simulink model "swing_up_test"  (R2020b)
settings: Solver=FixedStepDiscrete  StartTime=0.0  StopTime=Inf  FixedStep=0.001  MaxStep=0.001  RelTol=1e-3  EnableMultiTasking=on
values from neighbouring files (symbols this model uses):
  alfaBest = sin(2*pi*tacc/Tperiod)    [demo.m]    (also in pendulo_modelo.m)
  Xmax = 0.02    [demo.m]    (also in pendulo_modelo.m = 0.045)
  Xmin = -0.02    [demo.m]    (also in pendulo_modelo.m = -0.045)
libraries: simulink x3, arduinolib x2
settings Model: SILPILModeSetting=veronly  ExtModeTrigDuration=2  Creator=aleca  LastModifiedBy=aleca
settings OptimizationCC: EnhancedBackFolding=on  PassReuseOutputArgsAs=Individual arguments  ZeroExternalMemoryAtStartup=off  ZeroInternalMemoryAtStartup=off  MaxStackSize=64  OptimizeBlockOrder=speed  DifferentSizesBufferReuse=on  OptimizationCustomize=off  EfficientTunableParamExpr=on
settings DebuggingCC: ParameterTunabilityLossMsg=error
settings HardwareCC: ProdBitPerInt=16  ProdBitPerPointer=16  ProdBitPerSizeT=16  ProdBitPerPtrDiffT=16  ProdLargestAtomicFloat=None  ProdWordSize=8  ProdHWDeviceType=Atmel->AVR  UseEmbeddedCoderFeatures=off  UseSimulinkCoderFeatures=off
settings SFSimCC: MATLABDynamicMemAlloc=off
settings RTWCC: Description=Embedded Coder  SystemTargetFile=ert.tlc  HardwareBoard=Arduino Mega 2560  TemplateMakefile=ert_default_tmf  Toolchain=Arduino AVR  BuildConfiguration=Faster Runs
settings CodeAppCC: ForceParamTrailComments=on  IgnoreCustomStorageClasses=off  OperatorAnnotations=on  SimulinkDataObjDesc=on  SFDataObjDesc=on  InsertBlockDesc=on
settings ERTTargetCC: SupportContinuousTime=on  SupportNonInlinedSFcns=on  SupportVariableSizeSignals=on  ExtModeStaticAllocSize=2048

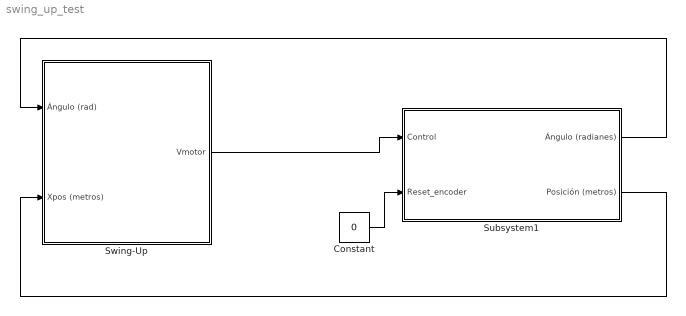
== system swing_up_test ==
  Constant : Constant  Value=0  OutDataTypeStr=boolean  SampleTime=-1
  Subsystem1 : Subsystem
  Swing-Up : Subsystem
  wires:
  Subsystem1/1(Ángulo (radianes)) -> Swing-Up/1(Ángulo (rad))
  Subsystem1/2(Posición (metros)) -> Swing-Up/2(Xpos (metros))
  Swing-Up/1(Vmotor) -> Subsystem1/1(Control)
  Constant/1 -> Subsystem1/2(Reset_encoder)

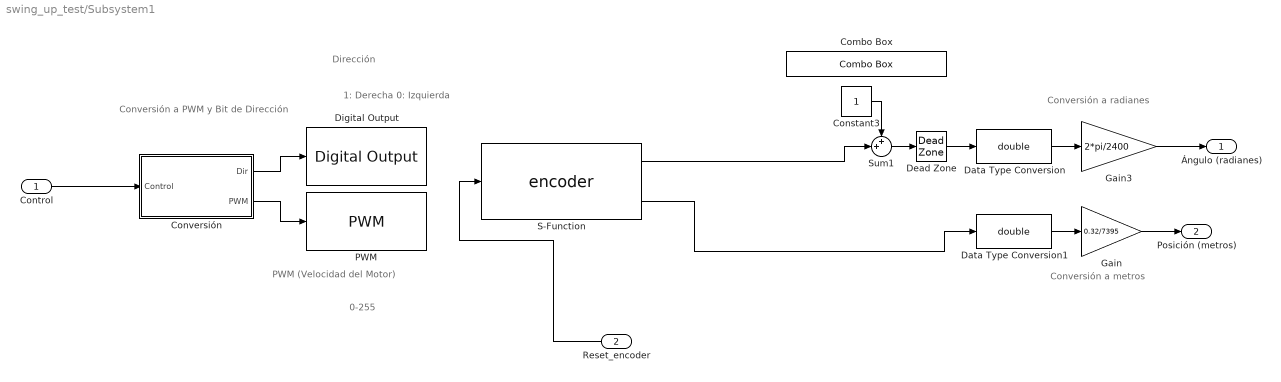
== system swing_up_test/Subsystem1 ==
  note: Conversión a metros
  note: Dirección
  note: PWM (Velocidad del Motor)
  note: 1: Derecha
      | 0: Izquierda
  note: Conversión a radianes
  note: 0-255
  note: Conversión a PWM y
      | Bit de Dirección
  Control : Inport
  Reset_encoder : Inport  Port=2
  Combo Box : ComboBox  LabelPosition=Hide  SelectedLabel=1
      settings: Values={{'0', '1', '2', '-2', '-1'}, [0 1 2 -2 -1]}
  Constant3 : Constant  SampleTime=-1
  Conversión : Subsystem
  Data Type Conversion : DataTypeConversion  OutDataTypeStr=double
  Data Type Conversion1 : DataTypeConversion  OutDataTypeStr=double
  Dead Zone : DeadZone  LowerValue=0  UpperValue=0  SaturateOnIntegerOverflow=on
  Digital Output : arduinolib/Digital Output  pinNumber=10  Direction=output  blockPlatform=arduino
  Gain : Gain  Gain=0.32/7395
  Gain3 : Gain  Gain=2*pi/2400
  PWM : arduinolib/PWM  pinNumber=9  frequencyType=Default  desiredFrequency=490.2  achievableFrequency=490.2
  S-Function : S-Function  FunctionName=encoder  SFunctionModules='encoder_wrapper'  SFunctionDeploymentMode=off  EnableBusSupport=off
  Sum1 : Sum  Inputs=++|
  Ángulo (radianes) : Outport
  Posición (metros) : Outport  Port=2
  wires:
  Gain/1 -> Posición (metros)/1
  Sum1/1 -> Dead Zone/1
  Conversión/1(Dir) -> Digital Output/1
  Conversión/2(PWM) -> PWM/1
  Dead Zone/1 -> Data Type Conversion/1
  Data Type Conversion/1 -> Gain3/1
  Constant3/1 -> Sum1/1
  S-Function/2 -> Data Type Conversion1/1
  Data Type Conversion1/1 -> Gain/1
  Reset_encoder/1 -> S-Function/1
  Control/1 -> Conversión/1(Control)
  Gain3/1 -> Ángulo (radianes)/1
  S-Function/1 -> Sum1/2

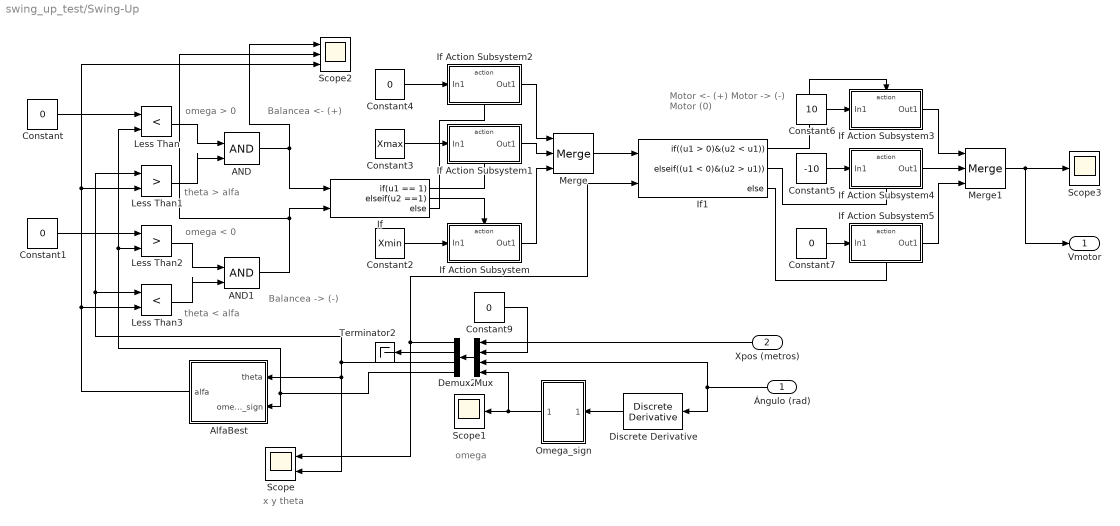
== system swing_up_test/Swing-Up ==
  note: x y theta
  note: omega
  note: Motor <- (+)
      | Motor -> (-)
      | Motor (0)
  note: Balancea -> (-)
  note: theta > alfa
  note: omega > 0
  note: omega < 0
  note: theta < alfa
  note: Balancea <- (+)
  Ángulo (rad) : Inport
  Xpos (metros) : Inport  Port=2
  AND : Logic  IconShape=distinctive  AllPortsSameDT=off  OutDataTypeStr=boolean
  AND1 : Logic  IconShape=distinctive  AllPortsSameDT=off  OutDataTypeStr=boolean
  AlfaBest : Subsystem
      settings: PortSchema="{\"entries\":[{\"content\":{\"sides\":[{\"content\":{\"connectorIds\":[\"Out1\"]},\"type\":\"ConnectorPlacement.EquallySpacedRectSide\",\"uuid\":\"f269d330-2dbf-4a03-aae2-9d91e46d5f46\"},{\"content\":{\"connectorIds\":[\"In1\",\"In2\"],\"side\":\"RIGHT\"},\"type\":\"ConnectorPlacement.EquallySpacedRectSide\",\"uuid\":\"83605d16-f426-4f00-b326-dfdad5d6c839\"},{\"content\":{\"connectorIds\":[],\"side\":\"TOP\"},\"type\":\"ConnectorPlacement.EquallySpacedRectSide\",\"uuid\":\"8003ed59-a4ef-474d-85bb-f26d1ffabd7e\"},{\"content\":{\"connectorIds\":[],\"side\":\"HIDDEN\"},\"type\":\"ConnectorPlacement.EquallySpacedRectSide\",\"uuid\":\"ae6ea9e2-c2fb-4e9e-9ec9-1e561a8d4724\"}]},\"type\":\"ConnectorPlacement.EquallySpacedConnector\",\"uuid\":\"f5174008-485c-4d77-9a7a-ef1ea74262ea\"}],\"packageUris\":[\"http://schema.mathworks.com/mf0/Connector/R2020b\"],\"version\":\"1.0\"}"
  Constant{,1,4,7} (4 alike) : Constant  Value=0  SampleTime=-1
  Constant2 : Constant  Value=Xmin  SampleTime=-1
  Constant3 : Constant  Value=Xmax  SampleTime=-1
  Constant5 : Constant  Value=-10  SampleTime=-1
  Constant6 : Constant  Value=10  SampleTime=-1
  Constant9 : Constant  Value=0
  Demux2 : Demux
  Discrete Derivative : simulink/Discrete/Discrete Derivative  gainval=1.0  ICPrevScaledInput=0.0  OutMin=[]  OutMax=[]  OutDataType=fixdt(1, 16)  OutScaling=2^-10  DoSatur=off
  If : If  NumInputs=2  IfExpression=u1 == 1  ElseIfExpressions=u2 ==1
  If Action Subsystem : Subsystem  TreatAsAtomicUnit=on
  If Action Subsystem1 : Subsystem  TreatAsAtomicUnit=on
  If Action Subsystem2 : Subsystem  TreatAsAtomicUnit=on
  If Action Subsystem3 : Subsystem  TreatAsAtomicUnit=on
  If Action Subsystem4 : Subsystem  TreatAsAtomicUnit=on
  If Action Subsystem5 : Subsystem  TreatAsAtomicUnit=on
  If1 : If  NumInputs=2  IfExpression=(u1 > 0)&(u2 < u1)  ElseIfExpressions=(u1 < 0)&(u2 > u1)
  Less Than : RelationalOperator  Operator=<  OutDataTypeStr=boolean  RndMeth=Simplest
  Less Than1 : RelationalOperator  Operator=>  OutDataTypeStr=boolean  RndMeth=Simplest
  Less Than2 : RelationalOperator  Operator=>  OutDataTypeStr=boolean  RndMeth=Simplest
  Less Than3 : RelationalOperator  Operator=<  OutDataTypeStr=boolean  RndMeth=Simplest
  Merge : Merge  Inputs=3
  Merge1 : Merge  Inputs=3
  Mux : Mux
  Omega_sign : Subsystem
  Scope : Scope  NumInputPorts=2
  Scope1 : Scope
  Scope2 : Scope  NumInputPorts=3
  Scope3 : Scope
  Terminator2 : Terminator
  Vmotor : Outport
  wires:
  Constant3/1 -> If Action Subsystem1/1(In1)
  Less Than1/1 -> AND/2
  AND1/1 -> If/2, Scope2/2
  Omega_sign/1(Out1) -> Scope1/1, Mux/4
  Less Than/1 -> AND/1
  If Action Subsystem5/1(Out1) -> Merge1/3
  Constant1/1 -> Less Than2/1
  Less Than2/1 -> AND1/1
  Constant/1 -> Less Than/1
  If Action Subsystem3/1(Out1) -> Merge1/1
  AND/1 -> Scope2/1, If/1
  Demux2/3 -> AlfaBest/1(theta), Scope/2, Less Than3/1, Less Than1/1
  Mux/1 -> Demux2/1
  If1/1 -> If Action Subsystem3/Action
  If Action Subsystem2/1(Out1) -> Merge/1
  Constant4/1 -> If Action Subsystem2/1(In1)
  Less Than3/1 -> AND1/2
  AlfaBest/1(alfa) -> Scope2/3, Less Than1/2, Less Than3/2
  Constant5/1 -> If Action Subsystem4/1(In1)
  Constant9/1 -> Mux/2
  Demux2/2 -> Terminator2/1
  Ángulo (rad)/1 -> Mux/3, Discrete Derivative/1
  Demux2/4 -> Less Than/2, Less Than2/2, AlfaBest/2(omega_sign)
  Demux2/1 -> Scope/1, If1/2
  Constant7/1 -> If Action Subsystem5/1(In1)
  If/2 -> If Action Subsystem/Action
  Constant2/1 -> If Action Subsystem/1(In1)
  Merge1/1 -> Vmotor/1, Scope3/1
  Constant6/1 -> If Action Subsystem3/1(In1)
  If1/3 -> If Action Subsystem5/Action
  If Action Subsystem/1(Out1) -> Merge/3
  If Action Subsystem4/1(Out1) -> Merge1/2
  Merge/1 -> If1/1
  Discrete Derivative/1 -> Omega_sign/1(In1)
  If/1 -> If Action Subsystem1/Action
  If/3 -> If Action Subsystem2/Action
  If Action Subsystem1/1(Out1) -> Merge/2
  If1/2 -> If Action Subsystem4/Action
  Xpos (metros)/1 -> Mux/1

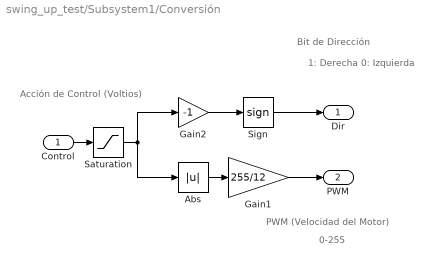
== system swing_up_test/Subsystem1/Conversión ==
  note: Acción de Control
      | (Voltios)
  note: Bit de Dirección
  note: 1: Derecha
      | 0: Izquierda
  note: 0-255
  note: PWM (Velocidad del Motor)
  Control : Inport
  Abs : Abs
  Gain1 : Gain  Gain=255/12
  Gain2 : Gain  Gain=-1
  Saturation : Saturate  UpperLimit=12  LowerLimit=-12
  Sign : Signum
  Dir : Outport
  PWM : Outport  Port=2
  wires:
  Abs/1 -> Gain1/1
  Gain1/1 -> PWM/1
  Control/1 -> Saturation/1
  Saturation/1 -> Gain2/1, Abs/1
  Sign/1 -> Dir/1
  Gain2/1 -> Sign/1

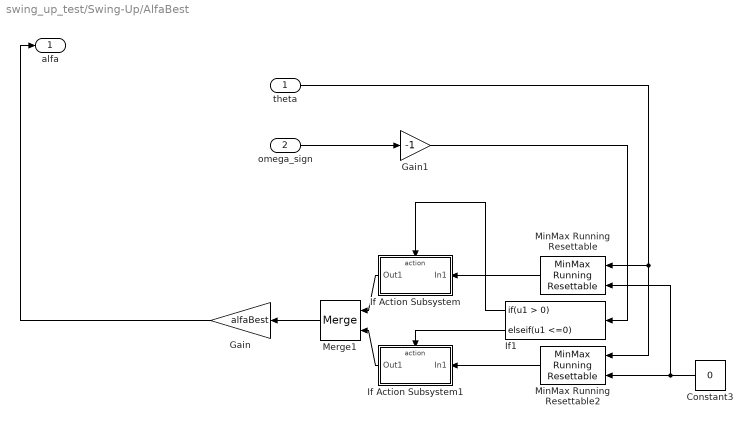
== system swing_up_test/Swing-Up/AlfaBest ==
  theta : Inport
  omega_sign : Inport  Port=2
  Constant3 : Constant  Value=0
  Gain : Gain  Gain=alfaBest
  Gain1 : Gain  Gain=-1
  If Action Subsystem : Subsystem  TreatAsAtomicUnit=on
  If Action Subsystem1 : Subsystem  TreatAsAtomicUnit=on
  If1 : If  ElseIfExpressions=u1 <=0  ShowElse=off
  Merge1 : Merge
  MinMax Running Resettable : simulink/Math Operations/MinMax Running Resettable  Function=max  vinit=0.0
  MinMax Running Resettable2 : simulink/Math Operations/MinMax Running Resettable  Function=min  vinit=0.0
  alfa : Outport
  wires:
  Constant3/1 -> MinMax Running Resettable/2, MinMax Running Resettable2/2
  If Action Subsystem1/1(Out1) -> Merge1/2
  theta/1 -> MinMax Running Resettable2/1, MinMax Running Resettable/1
  MinMax Running Resettable2/1 -> If Action Subsystem1/1(In1)
  If1/1 -> If Action Subsystem/Action
  Merge1/1 -> Gain/1
  Gain/1 -> alfa/1
  MinMax Running Resettable/1 -> If Action Subsystem/1(In1)
  If Action Subsystem/1(Out1) -> Merge1/1
  If1/2 -> If Action Subsystem1/Action
  omega_sign/1 -> Gain1/1
  Gain1/1 -> If1/1

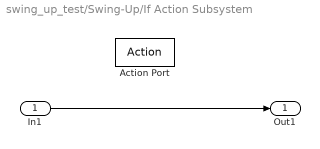
== system swing_up_test/Swing-Up/If Action Subsystem ==
  In1 : Inport
  Action Port : ActionPort  ActionPortLabel=elseif(u2 ==1)
  Out1 : Outport
  wires:
  In1/1 -> Out1/1

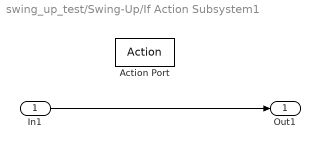
== system swing_up_test/Swing-Up/If Action Subsystem1 ==
  In1 : Inport
  Action Port : ActionPort  ActionPortLabel=if(u1 == 1)
  Out1 : Outport
  wires:
  In1/1 -> Out1/1

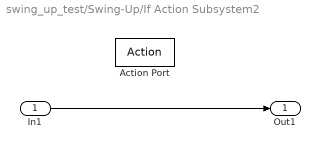
== system swing_up_test/Swing-Up/If Action Subsystem2 ==
  In1 : Inport
  Action Port : ActionPort  ActionPortLabel=else
  Out1 : Outport
  wires:
  In1/1 -> Out1/1

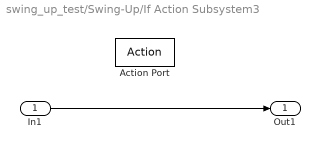
== system swing_up_test/Swing-Up/If Action Subsystem3 ==
  In1 : Inport
  Action Port : ActionPort  ActionPortLabel=if((u1 > 0)&(u2 < u1))
  Out1 : Outport
  wires:
  In1/1 -> Out1/1

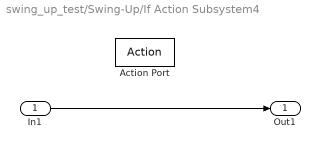
== system swing_up_test/Swing-Up/If Action Subsystem4 ==
  In1 : Inport
  Action Port : ActionPort  ActionPortLabel=elseif((u1 < 0)&(u2 > u1))
  Out1 : Outport
  wires:
  In1/1 -> Out1/1

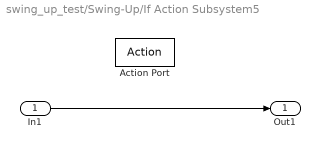
== system swing_up_test/Swing-Up/If Action Subsystem5 ==
  In1 : Inport
  Action Port : ActionPort  ActionPortLabel=else
  Out1 : Outport
  wires:
  In1/1 -> Out1/1

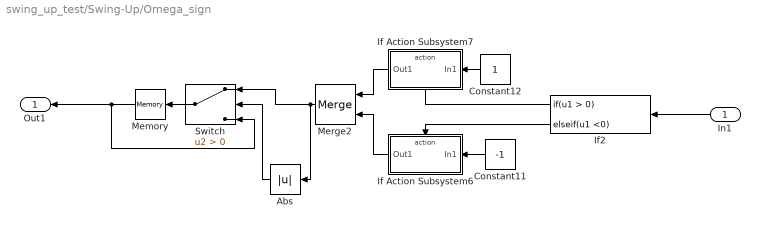
== system swing_up_test/Swing-Up/Omega_sign ==
  In1 : Inport
  Abs : Abs
  Constant11 : Constant  Value=-1  SampleTime=-1
  Constant12 : Constant  SampleTime=-1
  If Action Subsystem6 : Subsystem  TreatAsAtomicUnit=on
  If Action Subsystem7 : Subsystem  TreatAsAtomicUnit=on
  If2 : If  ElseIfExpressions=u1 <0  ShowElse=off
  Memory : Memory
  Merge2 : Merge
  Switch : Switch  Criteria=u2 > Threshold
  Out1 : Outport
  wires:
  In1/1 -> If2/1
  If Action Subsystem6/1(Out1) -> Merge2/2
  Merge2/1 -> Abs/1, Switch/1
  Abs/1 -> Switch/2
  If2/1 -> If Action Subsystem7/Action
  If Action Subsystem7/1(Out1) -> Merge2/1
  If2/2 -> If Action Subsystem6/Action
  Memory/1 -> Out1/1, Switch/3
  Switch/1 -> Memory/1
  Constant12/1 -> If Action Subsystem7/1(In1)
  Constant11/1 -> If Action Subsystem6/1(In1)

== system swing_up_test/Swing-Up/AlfaBest/If Action Subsystem ==
  In1 : Inport
  Action Port : ActionPort  ActionPortLabel=if(u1 > 0)
  Out1 : Outport
  wires:
  In1/1 -> Out1/1

== system swing_up_test/Swing-Up/AlfaBest/If Action Subsystem1 ==
  In1 : Inport
  Action Port : ActionPort  ActionPortLabel=elseif(u1 <=0)
  Out1 : Outport
  wires:
  In1/1 -> Out1/1

== system swing_up_test/Swing-Up/Omega_sign/If Action Subsystem6 ==
  In1 : Inport
  Action Port : ActionPort  ActionPortLabel=elseif(u1 <0)
  Out1 : Outport
  wires:
  In1/1 -> Out1/1

== system swing_up_test/Swing-Up/Omega_sign/If Action Subsystem7 ==
  In1 : Inport
  Action Port : ActionPort  ActionPortLabel=if(u1 > 0)
  Out1 : Outport
  wires:
  In1/1 -> Out1/1
